simulink library "calculateOptimalWingAngle"  (R2018a)
settings: Solver=VariableStepAuto  StartTime=0.0  StopTime=10.0  RelTol=1e-3
undefined symbols (not defined in the file): plant
settings Model: Creator=mitch  LastModifiedBy=M.Cobb

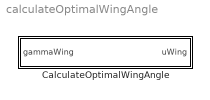
== system calculateOptimalWingAngle ==
  CalculateOptimalWingAngle : Subsystem

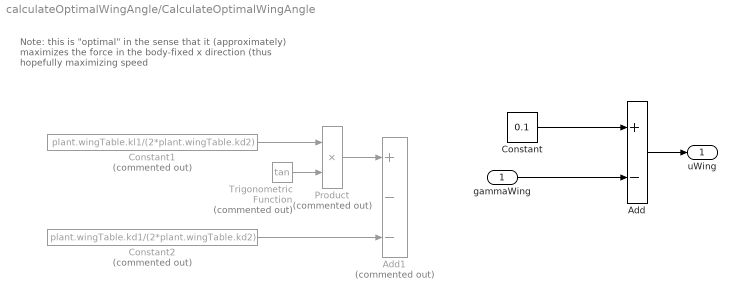
== system calculateOptimalWingAngle/CalculateOptimalWingAngle ==
  note: Note: this is "optimal" in the sense that it (approximately)
      | maximizes the force in the body-fixed x direction (thus
      | hopefully maximizing speed
  gammaWing : Inport  Unit=rad
  Add : Sum  Inputs=+-
  Add1 : Sum  Commented=on  Inputs=+--
  Constant : Constant  Value=0.1
  Constant1 : Constant  Commented=on  Value=plant.wingTable.kl1/(2*plant.wingTable.kd2)
  Constant2 : Constant  Commented=on  Value=plant.wingTable.kd1/(2*plant.wingTable.kd2)
  Product : Product  Commented=on
  Trigonometric Function : Trigonometry  Commented=on  Operator=tan
  uWing : Outport  Unit=rad
  wires:
  Constant2/1 -> Add1/3
  Constant1/1 -> Product/1
  Product/1 -> Add1/1
  Trigonometric Function/1 -> Product/2
  gammaWing/1 -> Add/2
  Constant/1 -> Add/1
  Add/1 -> uWing/1
